simulink subsystem "Drive_Servo"  (R2025b)
settings: Solver=VariableStepAuto  StartTime=0.0  StopTime=10.0  RelTol=1e-3
model mask{channel=2}
  mask prompts: channel "Servo Channel (0-15)"
libraries: raspberrypiCommlib x4
settings Model: Creator=Maken  LastModifiedBy=david

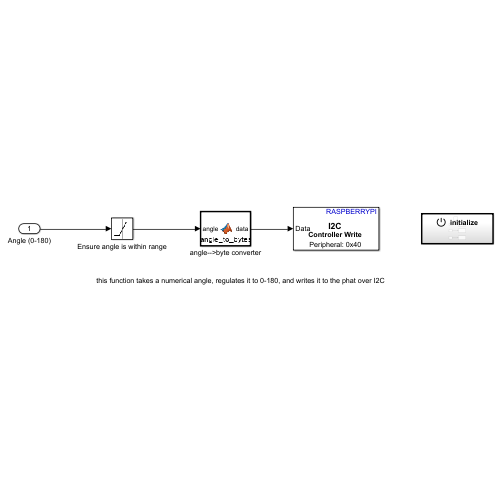
[thumbnail: Simulink's stored preview of the top-level diagram]
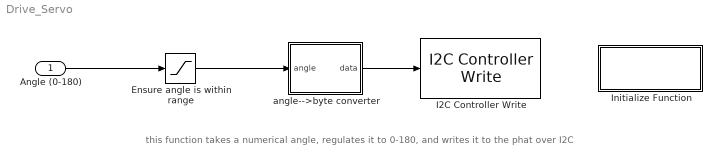
== system Drive_Servo ==
  note: this function takes a numerical angle, regulates it to 0-180, and writes it to the phat over I2C
  Angle (0-180) : Inport
  Ensure angle is within range : Saturate  UpperLimit=180  LowerLimit=0
  I2C Controller Write : raspberrypiCommlib/I2C Controller Write  BoardProperty=Pi 5 Model  I2CModule=1  Mode=Master  SlaveAddress=0x40  SlaveByteOrder=LittleEndian  Direction=Transmitter  RegisterAddressMode=on  RegisterAddress=0x06 + (channel * 4)  SlaveDataType=uint8  DataLength=1  NoAck=off  RepeatedStart=off  OutputStatus=off
  Initialize Function : Subsystem  TreatAsAtomicUnit=on
  angle-->byte converter : MATLAB Function  TreatAsAtomicUnit=on
  wires:
  angle-->byte converter/1(data) -> I2C Controller Write/1
  Angle (0-180)/1 -> Ensure angle is within range/1
  Ensure angle is within range/1 -> angle-->byte converter/1(angle)

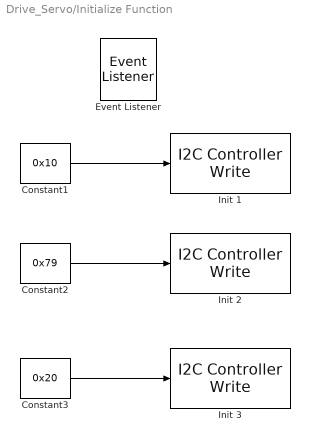
== system Drive_Servo/Initialize Function ==
  Constant1 : Constant  Value=0x10
  Constant2 : Constant  Value=0x79
  Constant3 : Constant  Value=0x20
  Event Listener : EventListener  DisableCoverage=on  EventName=reset
  Init 1 : raspberrypiCommlib/I2C Controller Write  BoardProperty=Pi 5 Model  I2CModule=1  Mode=Master  SlaveAddress=0x40  SlaveByteOrder=LittleEndian  Direction=Transmitter  RegisterAddressMode=on  RegisterAddress=0x00  SlaveDataType=uint8  DataLength=1  NoAck=off  RepeatedStart=off  OutputStatus=off
  Init 2 : raspberrypiCommlib/I2C Controller Write  BoardProperty=Pi 5 Model  I2CModule=1  Mode=Master  SlaveAddress=0x40  SlaveByteOrder=LittleEndian  Direction=Transmitter  RegisterAddressMode=on  RegisterAddress=0xFE  SlaveDataType=uint8  DataLength=1  NoAck=off  RepeatedStart=off  OutputStatus=off
  Init 3 : raspberrypiCommlib/I2C Controller Write  BoardProperty=Pi 5 Model  I2CModule=1  Mode=Master  SlaveAddress=0x40  SlaveByteOrder=LittleEndian  Direction=Transmitter  RegisterAddressMode=on  RegisterAddress=0x00  SlaveDataType=uint8  DataLength=1  NoAck=off  RepeatedStart=off  OutputStatus=off
  wires:
  Constant3/1 -> Init 3/1
  Constant2/1 -> Init 2/1
  Constant1/1 -> Init 1/1

== matlab function Drive_Servo/angle-->byte converter ==
  data: angle input; data output
function data = angle_to_bytes(angle)
%#codegen
angle_clamped = max(0.0, min(180.0, double(angle)));
tick = uint16(round(205 + (angle_clamped / 180.0) * 205));
off_l = uint8(bitand(tick, uint16(255)));
off_h = uint8(bitshift(tick, -8));
data = [uint8(0), uint8(0), off_l, off_h];
